simulink model "bd_par_auto2"  (Simulink 4.1.1)
settings: Solver=ode1  SolverMode=SingleTasking  StartTime=0.0  StopTime=max(cyc_mph(:,1))  FixedStep=1  MaxStep=1  RelTol=1e-3  AbsTol=1e-3
undefined symbols (not defined in the file): air_cp, amb_tmp, cs_charge_deplete_bool, cs_charge_trq, cs_electric_decel_spd, cs_electric_launch_spd_hi, cs_electric_launch_spd_lo, cs_hi_soc, cs_lo_soc, cs_min_trq_frac, cs_off_trq_frac, cyc_avg_time, cyc_cargo_mass, cyc_elevation_init, cyc_filter_bool, cyc_grade, cyc_mph, enable_stop, ess_cap_scale, ess_coulombic_eff, ess_init_soc, ess_max_ah_cap, ess_max_volts, ess_min_volts, ess_mod_airflow, ess_mod_cp, ess_mod_init_tmp, ess_module_mass, ess_module_num, ess_on, ess_res_scale_coef, ess_res_scale_fun, ess_set_tmp, ess_th_calc, ess_th_res_off, ess_th_res_on, ess_tmp, ess_voc, ex_calc, fc_ct_trq, fc_emis, fc_inertia, fc_map_spd, fc_max_trq, fc_on, fc_spd_scale, fc_trq_scale, fc_tstat, fd_inertia, fd_loss, fd_ratio, gb_dnshift_load, gb_dnshift_spd, gb_gears_num, gb_inertia, gb_num_init, gb_ratio, gb_shift_delay, gb_spd_scale, gb_trq_scale ... (+56)
libraries: lib_wheel2 x12, lib_accessory2 x3, lib_etc x2, lib_drive_cycle2 x1, lib_interactive x1, lib_drive_cycle x1, lib_exhaust x1, lib_fuel_converter3 x1
(part 17 of 18)

== system bd_par_auto2/fuel converter <fc>/IC Engine Model  &  Interface/ic engine model/engine torque/T_max ==
  w_APU : Inport  Port=1  LatchInput=off
  Saturation1 : Saturate  UpperLimit=max(fc_map_spd)*fc_spd_scale  LowerLimit=min(fc_map_spd)*fc_spd_scale  LinearizeAsGain=on
  max_torque lookup : Lookup  InputValues=fc_map_spd*fc_spd_scale  OutputValues=fc_max_trq*fc_trq_scale
  T_max : Outport  Port=1  InitialOutput=0
  tag scope: engine_speed=scoped
  wires:
  w_APU/1 -> Saturation1/1
  max_torque lookup/1 -> T_max/1
  Saturation1/1 -> max_torque lookup/1, [engine_speed]

== system bd_par_auto2/fuel converter <fc>/IC Engine Model  &  Interface/ic engine model/engine torque/effect of inertia (Nm) ==
  engine spd (rad/s) : Inport  Port=1  LatchInput=off
  >=0 : Saturate  UpperLimit=inf  LowerLimit=0  LinearizeAsGain=on
  Block NOTES : Subsystem
      settings: RTWFcnNameOpts=Auto  RTWFileNameOpts=Auto
      mask Display: disp('Block\nNOTES')
  Clock : Clock
      settings: DisplayTime=off  Decimation=10
  Constant : Constant  Orientation=left  Value=fc_inertia
  Constant1 : Constant  Value=max(fc_max_trq)*fc_trq_scale
  Constant2 : Constant  Orientation=left  Value=0.01
  Memory : Memory  X0=-0.1  InheritSampleTime=off
      settings: RTWStateStorageClass=Auto
  Memory1 : Memory  X0=vc_idle_spd*vc_key_on(1,2)  InheritSampleTime=off
      settings: RTWStateStorageClass=Auto
  MinMax : MinMax  Function=min  Inputs=2
  Product : Product  Inputs=2  Multiplication=Element-wise(.*)  SaturateOnIntegerOverflow=on
  Product1 : Product  Inputs=*/*  Multiplication=Element-wise(.*)  SaturateOnIntegerOverflow=on
  Relational : RelationalOperator  Operator=>
  Sum : Sum  Inputs=+-  SaturateOnIntegerOverflow=on
  Sum1 : Sum  Inputs=+-  SaturateOnIntegerOverflow=on
  Sum2 : Sum  Inputs=-+  SaturateOnIntegerOverflow=on
  Switch : Switch  Threshold=eps
  engine inertia as a function of total vehicle inertia (generous approximation) : Subsystem  Orientation=down
      settings: RTWFcnNameOpts=Auto  RTWFileNameOpts=Auto
  (Nm) : Outport  Port=1  InitialOutput=0
  wires:
  Sum/1 -> >=0/1, Switch/3
  Memory1/1 -> Sum/2
  Product/1 -> MinMax/1
  Constant1/1 -> Product/2
  engine inertia as a function of total vehicle inertia (generous approximation)/1(Out1) -> Product/1
  Product1/1 -> MinMax/2
  MinMax/1 -> (Nm)/1
  [cyc_mph_r_prev] -> Sum2/2
  [mpha_prev] -> Sum2/1
  Switch/1 -> Product1/1
  Sum1/1 -> Product1/2
  Constant/1 -> Product1/3
  Memory/1 -> Sum1/2
  Clock/1 -> Memory/1, Sum1/1
  Relational/1 -> Switch/2
  >=0/1 -> Switch/1
  Sum2/1 -> Relational/1
  Constant2/1 -> Relational/2
  engine spd (rad/s)/1 -> Memory1/1, Sum/1

== system bd_par_auto2/gearbox <gb> old/gearbox model & interface/gearbox model/Pout/Pin neglecting inertia/Pout/Pin (neglecting inertia) ==
  in_1 : Inport  Port=1  LatchInput=off
  in_2 : Inport  Port=2  LatchInput=off
  Fcn : Fcn  Expr=1/u
  Product : Product  Inputs=2  Multiplication=Element-wise(.*)  SaturateOnIntegerOverflow=on
  out_1 : Outport  Port=1  InitialOutput=0
  wires:
  in_1/1 -> Product/1
  Fcn/1 -> Product/2
  Product/1 -> out_1/1
  in_2/1 -> Fcn/1

== system bd_par_auto2/gearbox <gb> old/gearbox model & interface/gearbox model/Pout/Pin neglecting inertia/make division bombproof ==
  note: only add eps if Tin-Tinertia is == 0 (this avoids problems when Tin-Tineratia == -eps
      | which happens from time to time
  Tin-Tinertia : Inport  Port=1  LatchInput=off
  Block NOTES : Subsystem
      settings: RTWFcnNameOpts=Auto  RTWFileNameOpts=Auto
      mask Display: disp('Block\nNOTES')
  Constant : Constant  Orientation=up  Value=eps
  Constant1 : Constant  Orientation=up  Value=0
  Product : Product  Inputs=2  Multiplication=Element-wise(.*)  SaturateOnIntegerOverflow=on
  Relational Operator1 : RelationalOperator  Operator===
  make division bombproof : Sum  Inputs=++  SaturateOnIntegerOverflow=on
  Out1 : Outport  Port=1
  wires:
  Tin-Tinertia/1 -> make division bombproof/1, Relational Operator1/1
  Constant1/1 -> Relational Operator1/2
  Product/1 -> make division bombproof/2
  Relational Operator1/1 -> Product/1
  Constant/1 -> Product/2
  make division bombproof/1 -> Out1/1

== system bd_par_auto2/gearbox <gb> old/gearbox model & interface/gearbox model/gearbox controller interface/enhancedToWorkspace1 ==
  In1 : Inport  Port=1  LatchInput=off
  Terminator : Terminator
  wires:
  In1/1 -> Terminator/1

== system bd_par_auto2/gearbox <gb> old/gearbox model & interface/gearbox model/gearbox controller interface/enhancedToWorkspace8 ==
  In1 : Inport  Port=1  LatchInput=off
  Terminator : Terminator
  wires:
  In1/1 -> Terminator/1

== system bd_par_auto2/gearbox <gb> old/gearbox model & interface/gearbox model/loss (Nm)/3D discrete lookup table (sfun) ==
  lookup speed (rad/s) : Inport  Port=1  LatchInput=off
  lookup trq (Nm) : Inport  Port=2  LatchInput=off
  "gear_number  (e.g., 1, 2, 3)" : Inport  Port=3  LatchInput=off
  Mux : Mux  Inputs=3
  Saturation : Saturate  UpperLimit=max(tx_map_spd)  LowerLimit=min(tx_map_spd)  LinearizeAsGain=on
  Saturation1 : Saturate  UpperLimit=max(tx_map_trq)  LowerLimit=min(tx_map_trq)  LinearizeAsGain=on
  Saturation2 : Saturate  UpperLimit=size(tx_eff_map,3)  LowerLimit=1  LinearizeAsGain=on
  discrete interp2d : S-Function  FunctionName=sfun_discreteLookup3d  Parameters=tx_map_trq, tx_map_spd, tx_eff_map  PortCounts=[]  SFunctionModules=''
  tx_eff : Outport  Port=1
  wires:
  Saturation2/1 -> Mux/3
  "gear_number  (e.g., 1, 2, 3)"/1 -> Saturation2/1
  Saturation1/1 -> Mux/2
  lookup trq (Nm)/1 -> Saturation1/1
  Saturation/1 -> Mux/1
  lookup speed (rad/s)/1 -> Saturation/1
  Mux/1 -> discrete interp2d/1
  discrete interp2d/1 -> tx_eff/1

== system bd_par_auto2/gearbox <gb> old/gearbox model & interface/gearbox model/loss (Nm)/Block NOTES ==
  note: Revision Notes:
  note: 09/20/02:tm modifed lower input to switch after T_loss_at_input to pass the
      | total torque input as the loss when tx_eff=0
      | 5 July 2001:mpo changing loss block to a lookup table methodology
      | 12/20/00:tm revised loss saturation block. lower limit changed
      | from 1 to 0 and upper limit changed from 100 to inf to prevent over or under penalties

== system bd_par_auto2/gearbox <gb> old/gearbox model & interface/gearbox model/loss (Nm)/enhancedToWorkspace ==
  In1 : Inport  Port=1  LatchInput=off
  Terminator : Terminator
  wires:
  In1/1 -> Terminator/1

== system bd_par_auto2/hydraulic torque converter <htc> HEV/HTC for parallel HEV and Interface/model for parallel HEV/SR/K_adv ==
  "Req'd output trq and spd (Nm), (rad/s)" : Inport  Port=1  LatchInput=off
  >0 : Saturate  UpperLimit=inf  LowerLimit=eps  LinearizeAsGain=on
  K_adv=wout/(Tout)^0.5 : Fcn  Expr=u[2]/u[1]^0.5
  Saturation : Saturate  UpperLimit=max(htc_k_adv)  LowerLimit=min(htc_k_adv)  LinearizeAsGain=on
  K_adv : Outport  Port=1
  wires:
  Saturation/1 -> K_adv/1
  K_adv=wout/(Tout)^0.5/1 -> Saturation/1
  "Req'd output trq and spd (Nm), (rad/s)"/1 -> >0/1
  >0/1 -> K_adv=wout/(Tout)^0.5/1

== system bd_par_auto2/hydraulic torque converter <htc> HEV/HTC for parallel HEV and Interface/model for parallel HEV/SR/K_adv_coast ==
  "Req'd output trq and spd (Nm), (rad/s)" : Inport  Port=1  LatchInput=off
  K_adv=wout/(abs(Tout))^0.5 : Fcn  Expr=u[2]/abs(u[1]+eps)^0.5
  Saturation : Saturate  UpperLimit=max(htc_k_adv_coast)  LowerLimit=0  LinearizeAsGain=on
  K_adv_coast : Outport  Port=1
  wires:
  "Req'd output trq and spd (Nm), (rad/s)"/1 -> K_adv=wout/(abs(Tout))^0.5/1
  Saturation/1 -> K_adv_coast/1
  K_adv=wout/(abs(Tout))^0.5/1 -> Saturation/1

== system bd_par_auto2/hydraulic torque converter <htc> HEV/HTC for parallel HEV and Interface/model for parallel HEV/SR/enhancedToWorkspace ==
  In1 : Inport  Port=1  LatchInput=off
  To Workspace : ToWorkspace  VariableName=htc_locked  SampleTime=-1  SaveFormat=Array
  wires:
  In1/1 -> To Workspace/1

== system bd_par_auto2/hydraulic torque converter <htc> HEV/HTC for parallel HEV and Interface/model for parallel HEV/SR/enhancedToWorkspace1 ==
  In1 : Inport  Port=1  LatchInput=off
  To Workspace : ToWorkspace  VariableName=htc_coasting  SampleTime=-1  SaveFormat=Array
  wires:
  In1/1 -> To Workspace/1

== system bd_par_auto2/hydraulic torque converter <htc> HEV/HTC for parallel HEV and Interface/model for parallel HEV/SR/shifting SR ==
  T,w req out : Inport  Port=1  LatchInput=off
  w in : Inport  Port=2  LatchInput=off
  SR : Inport  Port=3  LatchInput=off
  -3200 rpm/second allowable in engine speed : Gain  Gain=-3200*pi/30  Multiplication=Element-wise(K.*u)  SaturateOnIntegerOverflow=on
  >0 : Saturate  UpperLimit=inf  LowerLimit=eps  LinearizeAsGain=on
  Clock : Clock
      settings: DisplayTime=off  Decimation=10
  Memory3 : Memory  X0=eps  InheritSampleTime=off
      settings: RTWStateStorageClass=Auto
  Memory4 : Memory  X0=0  InheritSampleTime=off
      settings: RTWStateStorageClass=Auto
  MinMax : MinMax  Function=min  Inputs=2
  SRmax= wout/win,min : Product  Inputs=*/  Multiplication=Element-wise(.*)  SaturateOnIntegerOverflow=on
  dt=t-(t-1) : Sum  Inputs=+-  SaturateOnIntegerOverflow=on
  "shifting, then limit  engine speed change" : Switch  Threshold=eps
  win,min= win,prev+rate*dt : Sum  Inputs=++  SaturateOnIntegerOverflow=on
  wout,req : Selector  InputType=Vector  ElementSrc=Internal  Elements=2  RowSrc=Internal  Rows=1  ColumnSrc=Internal  Columns=1  InputPortWidth=2
  SR limited : Outport  Port=1  InitialOutput=0
  wires:
  Memory4/1 -> dt=t-(t-1)/2
  Clock/1 -> Memory4/1, dt=t-(t-1)/1
  dt=t-(t-1)/1 -> -3200 rpm/second allowable in engine speed/1
  Memory3/1 -> win,min= win,prev+rate*dt/1
  win,min= win,prev+rate*dt/1 -> SRmax= wout/win,min/2
  wout,req/1 -> SRmax= wout/win,min/1
  T,w req out/1 -> wout,req/1
  [shifting] -> "shifting, then limit  engine speed change"/2
  SRmax= wout/win,min/1 -> MinMax/1
  SR/1 -> "shifting, then limit  engine speed change"/3, MinMax/2
  "shifting, then limit  engine speed change"/1 -> SR limited/1
  MinMax/1 -> "shifting, then limit  engine speed change"/1
  w in/1 -> >0/1
  >0/1 -> Memory3/1
  -3200 rpm/second allowable in engine speed/1 -> win,min= win,prev+rate*dt/2

== system bd_par_auto2/hydraulic torque converter <htc> HEV/HTC for parallel HEV and Interface/model for parallel HEV/T, shifting/T_max ==
  w_APU : Inport  Port=1  LatchInput=off
  TR : Inport  Port=2  LatchInput=off
  Block NOTES : Subsystem
      settings: RTWFcnNameOpts=Auto  RTWFileNameOpts=Auto
      mask Display: disp('Block\nNOTES')
  Constant : Constant  Value=1
  Gain : Gain  Gain=tc_mc_to_fc_ratio  Multiplication=Element-wise(K.*u)  SaturateOnIntegerOverflow=on
  Gain1 : Gain  Gain=tc_mc_to_fc_ratio  Multiplication=Element-wise(K.*u)  SaturateOnIntegerOverflow=on
  Saturation1 : Saturate  UpperLimit=max(fc_map_spd)*fc_spd_scale  LowerLimit=min(fc_map_spd)*fc_spd_scale  LinearizeAsGain=on
  Sum : Sum  Inputs=++  SaturateOnIntegerOverflow=on
  Switch : Switch  Threshold=eps
  Tin*TR= Tout : Product  Inputs=2  Multiplication=Element-wise(.*)  SaturateOnIntegerOverflow=on
  max_torque  mc lookup1 : Lookup  InputValues=mc_map_spd*mc_spd_scale  OutputValues=mc_max_trq*mc_overtrq_factor*mc_trq_scale
  max_torque lookup : Lookup  InputValues=fc_map_spd*fc_spd_scale  OutputValues=fc_max_trq*fc_trq_scale
  T_max max gain from htc : Outport  Port=1  InitialOutput=0
  wires:
  w_APU/1 -> Saturation1/1
  Tin*TR= Tout/1 -> T_max max gain from htc/1
  TR/1 -> Tin*TR= Tout/2
  max_torque lookup/1 -> Sum/1
  Saturation1/1 -> max_torque lookup/1, Gain/1
  Gain/1 -> max_torque  mc lookup1/1
  max_torque  mc lookup1/1 -> Gain1/1
  Constant/1 -> Switch/2
  Sum/1 -> Switch/1
  Gain1/1 -> Sum/2, Switch/3
  Switch/1 -> Tin*TR= Tout/1

== system bd_par_auto2/hydraulic torque converter <htc> HEV/HTC for parallel HEV and Interface/model for parallel HEV/T, shifting/engine speed estimator ==
  htc_spd_in_a : Inport  Port=1  LatchInput=off
  Memory2 : Memory  X0=0  InheritSampleTime=off
      settings: RTWStateStorageClass=Auto
  Out1 : Outport  Port=1
  wires:
  htc_spd_in_a/1 -> Memory2/1
  Memory2/1 -> Out1/1

== system bd_par_auto2/motor/controller <mc>/motor model & interface/mc model/N-m drive torque per W input/Block NOTES ==
  note: This block determines the ratio of req'd rotor torque to req'd electrical input power,
      |  which is proportional to efficiency if the motor is providing torque.  This ratio is used
      | to compute actual rotor torque given some input power which may be different from
      | the req'd value.
      |
      | If the denominator, the req'd input power, is zero, this block outputs inf,
      | which is a flag used by the block .../rotor drive torque available (Nm).

== system bd_par_auto2/motor/controller <mc>/motor model & interface/mc model/effect of inertia (Nm)/Block NOTES ==
  note: Torque required to accelerate the motor's inertia is calculated from the rate of change
      | of mc_spd_out_a.  It is no greater than the product of the maximum motor torque and
      | the fractional contribution of the motor's inertia to the total vehicle inertia.

== system bd_par_auto2/motor/controller <mc>/motor model & interface/mc model/effect of inertia (Nm)/motor inertia as a function of total vehicle inertia (generous approximation) ==
  gear ratio : Inport  Orientation=down  Port=1  LatchInput=off
  Product : Product  Orientation=down  Inputs=*/  Multiplication=Element-wise(.*)  SaturateOnIntegerOverflow=on
  Sum : Sum  Orientation=down  Inputs=++|  SaturateOnIntegerOverflow=on
  engine inertia as a fraction of total vehicle inertia  (generous approximation)--denomenator : Fcn  Orientation=down  Expr=mc_inertia*u^2
  engine inertia as a fraction of total vehicle inertia  (generous approximation)--numerator : Fcn  Orientation=down  Expr=mc_inertia*u^2
  Out1 : Outport  Orientation=down  Port=1
  wires:
  Sum/1 -> Product/2
  engine inertia as a fraction of total vehicle inertia  (generous approximation)--denomenator/1 -> Sum/2
  [current_veh_mass] -> Sum/1
  gear ratio/1 -> engine inertia as a fraction of total vehicle inertia  (generous approximation)--denomenator/1, engine inertia as a fraction of total vehicle inertia  (generous approximation)--numerator/1
  Product/1 -> Out1/1
  engine inertia as a fraction of total vehicle inertia  (generous approximation)--numerator/1 -> Product/1

== system bd_par_auto2/motor/controller <mc>/motor model & interface/mc model/enforce torque limit/Block NOTES ==
  note: This block enforces the maximum torque production and absorption
      | capability limits of the motor.  It assumes that exactly as much torque
      | can be absorbed as can be produced at a given speed.

== system bd_par_auto2/motor/controller <mc>/motor model & interface/mc model/enforce torque limit/enhancedToWorkspace ==
  In1 : Inport  Port=1  LatchInput=off
  To Workspace : ToWorkspace  VariableName=mc_max_trq_vec  SampleTime=-1  SaveFormat=Array
  wires:
  In1/1 -> To Workspace/1

== system bd_par_auto2/motor/controller <mc>/motor model & interface/mc model/mc tmp/Block NOTES ==
  note: This block models the thermal behavior of a motor
      | and controller  with active fluid cooling.
      | The module is modeled as a single lumped thermal mass.
      | The fan is on whenever the battery temp is > the set temp.

== system bd_par_auto2/motor/controller <mc>/motor model & interface/mc model/mc tmp/mc coolant ==
  Tcl : Inport  Port=1  LatchInput=off
  "Qmc " : Inport  Port=2  LatchInput=off
  Enable : EnablePort  StatesWhenEnabling=reset
  Constant : Constant  Value=mc_tstat
  Product1 : Product  Inputs=2  Multiplication=Element-wise(.*)  SaturateOnIntegerOverflow=on
  Relational Operator : RelationalOperator  Operator=<=
  Qmc_clt : Outport  Port=1  OutputWhenDisabled=reset  InitialOutput=0
  wires:
  Tcl/1 -> Relational Operator/2
  Constant/1 -> Relational Operator/1
  "Qmc "/1 -> Product1/2
  Product1/1 -> Qmc_clt/1
  Relational Operator/1 -> Product1/1

== system bd_par_auto2/motor/controller <mc>/motor model & interface/mc model/motor controller logic interface/motor controller logic ==
  bus voltage  previous : Inport  Port=1  LatchInput=off
  req'd input power (W) : Inport  Port=2  LatchInput=off
  req'd output spd (rad/s) : Inport  Port=3  LatchInput=off
  shifting : Inport  Port=4  LatchInput=off
  Abs : Abs  SaturateOnIntegerOverflow=on
  Abs1 : Abs  SaturateOnIntegerOverflow=on
  Block NOTES : Subsystem
      settings: RTWFcnNameOpts=Auto  RTWFileNameOpts=Auto
      mask Display: disp('Block\nNOTES')
  Constant : Constant  Value=mc_max_crrnt
  Constant1 : Constant  Value=0.001
  Constant2 : Constant  Orientation=left  Value=0
  Logical Operator1 : Logic  Orientation=up  Operator=NOT  Inputs=1
  MinMax : MinMax  Function=min  Inputs=2
  Product1 : Product  Inputs=2  Multiplication=Element-wise(.*)  SaturateOnIntegerOverflow=on
  Relational Operator : RelationalOperator  Operator=<=
  Relational Operator2 : RelationalOperator  Operator===
  Sign : Subsystem
      settings: RTWFcnNameOpts=Auto  RTWFileNameOpts=Auto
      mask Type: Sign
      mask Description: y = sign(x)
      mask Help: Sign Function:\n\t\t\ty = 1 if x > 0\n\t\t\ty = 0 if x = 0\n\t\t\ty = -1 if x < 0
      mask Display: plot(-50,-50,50,50,[-50,50],[0,0],[0,0],[-50,50],[-40,0],[-30,-30],[0,40],[30,30])
  Switch : Switch  Threshold=eps
  current-limited power : Product  Inputs=2  Multiplication=Element-wise(.*)  SaturateOnIntegerOverflow=on
  true if motor should be shut down : Logic  Operator=OR  Inputs=2
  req'd input power (W)1 : Outport  Port=1  InitialOutput=0
  tag scope: mc_crrnt_limited=scoped
  wires:
  shifting/1 -> true if motor should be shut down/2
  Logical Operator1/1 -> Switch/2
  true if motor should be shut down/1 -> Logical Operator1/1
  bus voltage  previous/1 -> Product1/1
  Constant/1 -> Product1/2
  req'd input power (W)/1 -> Abs/1, Sign/1(in_1)
  Abs/1 -> MinMax/2
  Sign/1(out_1) -> current-limited power/2
  Constant2/1 -> Switch/3
  Switch/1 -> req'd input power (W)1/1
  current-limited power/1 -> Switch/1
  Product1/1 -> MinMax/1, Relational Operator2/1
  MinMax/1 -> current-limited power/1, Relational Operator2/2
  Relational Operator2/1 -> [mc_crrnt_limited]
  Relational Operator/1 -> true if motor should be shut down/1
  Constant1/1 -> Relational Operator/2
  req'd output spd (rad/s)/1 -> Abs1/1
  Abs1/1 -> Relational Operator/1

== system bd_par_auto2/motor/controller <mc>/motor model & interface/mc model/motor speed estimator/Block NOTES ==
  note: The requested motor speed is replaced by an estimate of the
      | motor's previous speed, for loss and max. torque calculations,
      | whenever the vehicle missed the trace by more than 1 mph
      | on the last time step.

== system bd_par_auto2/motor/controller <mc>/motor model & interface/mc model/motor speed estimator/enhancedToWorkspace ==
  In1 : Inport  Port=1  LatchInput=off
  To Workspace : ToWorkspace  VariableName=mc_spd_est  SampleTime=-1  SaveFormat=Array
  wires:
  In1/1 -> To Workspace/1

== system bd_par_auto2/motor/controller <mc>/motor model & interface/mc model/motor speed estimator/init via port ==
  signal in : Inport  Port=1  LatchInput=off
  signal init : Inport  Port=2  LatchInput=off
  Constant : Constant  Value=1
  IC : InitialCondition  Value=0
  Switch : Switch  Threshold=0.5
  signal out : Outport  Port=1
  wires:
  signal init/1 -> Switch/3
  Switch/1 -> signal out/1
  IC/1 -> Switch/2
  Constant/1 -> IC/1
  signal in/1 -> Switch/1

== system bd_par_auto2/motor/controller <mc>/motor model & interface/mc model/rotor drive torque available (Nm)/Block NOTES ==
  note: This block computes the actual rotor torque given the actual motor input power and
      | the ratio (req'd rotor torque)/(req'd input power).
      |
      | If the above ratio has the value inf, which implies that the req'd input power is zero,
      | then the actual rotor torque is assumed to be zero.  This is not reflective of reality, of course:
      | with zero input power, the rotor torque would be the motor spin-loss torque at the given speed.
      | Because this simplification occurs only when req'd input power is zero, it does not.
      | affect fuel economy or max effort acceleration calculations.

== system bd_par_auto2/vehicle, wheel, & axle front/rear <wh> 2 axle --> 1 driveline/models and interface/vehicle <veh>/power logging--achieved/Joules ==
  In1 : Inport  Port=1  LatchInput=off
  To Workspace : ToWorkspace  VariableName=veh_energy_a  SampleTime=-1  SaveFormat=Array
  wires:
  In1/1 -> To Workspace/1

== system bd_par_auto2/vehicle, wheel, & axle front/rear <wh> 2 axle --> 1 driveline/models and interface/vehicle <veh>/power logging--achieved/horse power ==
  In1 : Inport  Port=1  LatchInput=off
  To Workspace : ToWorkspace  VariableName=veh_pwr_a_hp  SampleTime=-1  SaveFormat=Array
  wires:
  In1/1 -> To Workspace/1

== system bd_par_auto2/vehicle, wheel, & axle front/rear <wh> 2 axle --> 1 driveline/models and interface/vehicle <veh>/power logging--achieved/watts ==
  In1 : Inport  Port=1  LatchInput=off
  To Workspace : ToWorkspace  VariableName=veh_pwr_a  SampleTime=-1  SaveFormat=Array
  wires:
  In1/1 -> To Workspace/1

== system bd_par_auto2/vehicle, wheel, & axle front/rear <wh> 2 axle --> 1 driveline/models and interface/vehicle <veh>/power logging--request/Joules ==
  In1 : Inport  Port=1  LatchInput=off
  To Workspace : ToWorkspace  VariableName=veh_energy_r  SampleTime=-1  SaveFormat=Array
  wires:
  In1/1 -> To Workspace/1

== system bd_par_auto2/vehicle, wheel, & axle front/rear <wh> 2 axle --> 1 driveline/models and interface/vehicle <veh>/power logging--request/horse power ==
  In1 : Inport  Port=1  LatchInput=off
  To Workspace : ToWorkspace  VariableName=veh_pwr_r_hp  SampleTime=-1  SaveFormat=Array
  wires:
  In1/1 -> To Workspace/1

== system bd_par_auto2/vehicle, wheel, & axle front/rear <wh> 2 axle --> 1 driveline/models and interface/vehicle <veh>/power logging--request/watts ==
  In1 : Inport  Port=1  LatchInput=off
  To Workspace : ToWorkspace  VariableName=veh_pwr_r  SampleTime=-1  SaveFormat=Array
  wires:
  In1/1 -> To Workspace/1

== system bd_par_auto2/vehicle, wheel, & axle front/rear <wh> 2 axle --> 1 driveline/models and interface/vehicle <veh>/record achieved force outputs/enhancedToWorkspace ==
  In1 : Inport  Port=1  LatchInput=off
  To Workspace : ToWorkspace  VariableName=veh_pwr_accel_a  SampleTime=-1  SaveFormat=Array
  wires:
  In1/1 -> To Workspace/1

== system bd_par_auto2/vehicle, wheel, & axle front/rear <wh> 2 axle --> 1 driveline/models and interface/vehicle <veh>/record achieved force outputs/enhancedToWorkspace1 ==
  In1 : Inport  Port=1  LatchInput=off
  To Workspace : ToWorkspace  VariableName=veh_pwr_drag_a  SampleTime=-1  SaveFormat=Array
  wires:
  In1/1 -> To Workspace/1

== system bd_par_auto2/vehicle, wheel, & axle front/rear <wh> 2 axle --> 1 driveline/models and interface/vehicle <veh>/record achieved force outputs/enhancedToWorkspace2 ==
  In1 : Inport  Port=1  LatchInput=off
  To Workspace : ToWorkspace  VariableName=veh_pwr_ascent_a  SampleTime=-1  SaveFormat=Array
  wires:
  In1/1 -> To Workspace/1

== system bd_par_auto2/vehicle, wheel, & axle front/rear <wh> 2 axle --> 1 driveline/models and interface/vehicle <veh>/record achieved force outputs/enhancedToWorkspace3 ==
  In1 : Inport  Port=1  LatchInput=off
  To Workspace : ToWorkspace  VariableName=veh_pwr_rr_a  SampleTime=-1  SaveFormat=Array
  wires:
  In1/1 -> To Workspace/1

== system bd_par_auto2/vehicle, wheel, & axle front/rear <wh> 2 axle --> 1 driveline/models and interface/vehicle <veh>/record achieved force outputs/rolling resistance force ==
  average vehicle speed over time step (m/s) : Inport  Port=1  LatchInput=off
  force req'd to overcome rolling resistance (N) : lib_wheel2/Submodels/force req'd to overcome rolling resistance (N)
      settings: RTWFcnNameOpts=Auto  RTWFileNameOpts=Auto
  Fr (N) : Outport  Port=1
  wires:
  average vehicle speed over time step (m/s)/1 -> force req'd to overcome rolling resistance (N)/1
  force req'd to overcome rolling resistance (N)/1 -> Fr (N)/1

== system bd_par_auto2/vehicle, wheel, & axle front/rear <wh> 2 axle --> 1 driveline/models and interface/wheel and axle  front/rear <wh>/front force/brake request  controller interface ==
  F_front_brake_req : Outport  Port=1  InitialOutput=0
  wires:
  [F_front_brake_req] -> F_front_brake_req/1

== system bd_par_auto2/vehicle, wheel, & axle front/rear <wh> 2 axle --> 1 driveline/models and interface/wheel and axle  front/rear <wh>/front force/enhancedToWorkspace11 ==
  In1 : Inport  Port=1  LatchInput=off
  To Workspace : ToWorkspace  VariableName=wh_front_brake_r  SampleTime=-1  SaveFormat=Array
  wires:
  In1/1 -> To Workspace/1

== system bd_par_auto2/vehicle, wheel, & axle front/rear <wh> 2 axle --> 1 driveline/models and interface/wheel and axle  front/rear <wh>/limits and losses diagnostics/enhancedToWorkspace ==
  In1 : Inport  Port=1  LatchInput=off
  To Workspace : ToWorkspace  VariableName=wh_brake_loss_pwr  SampleTime=-1  SaveFormat=Array
  wires:
  In1/1 -> To Workspace/1

== system bd_par_auto2/vehicle, wheel, & axle front/rear <wh> 2 axle --> 1 driveline/models and interface/wheel and axle  front/rear <wh>/rear force/brake request controller interface1 ==
  F_rear_brake_req : Outport  Port=1  InitialOutput=0
  wires:
  [F_rear_brake_req] -> F_rear_brake_req/1

== system bd_par_auto2/vehicle, wheel, & axle front/rear <wh> 2 axle --> 1 driveline/models and interface/wheel and axle  front/rear <wh>/rear force/enhancedToWorkspace ==
  In1 : Inport  Port=1  LatchInput=off
  To Workspace : ToWorkspace  VariableName=wh_rear_brake_r  SampleTime=-1  SaveFormat=Array
  wires:
  In1/1 -> To Workspace/1

== system bd_par_auto2/vehicle, wheel, & axle front/rear <wh> 2 axle --> 1 driveline/models and interface/wheel and axle  front/rear <wh>/tire slip model (m/s)/Block NOTES ==
  note: This block implements the effects of finite tire slip (with respect to the road) on the
      | vehicle speed/wheel speed relationship.  Slip is defined as s=(omega*r - v) / v.  The
      | one-to-one mapping of slip to normalized tractive force, F_tract/W_front_axle, up to
      | the maximum, is stored in the variables "wh_slip" and "wh_slip_force_coeff."  The
      | slip calculation here is overridden if the actual axle speed and the requested axle
      | speed are the same, indicating that no drivetrain speed limits were encountered.

== system bd_par_auto2/vehicle, wheel, & axle front/rear <wh> 2 axle --> 1 driveline/models and interface/wheel and axle  front/rear <wh>/tire slip model (m/s)/front axle ==
  In1 : Inport  Port=1  LatchInput=off
  In2 : Inport  Port=2  LatchInput=off
  Abs : Abs  SaturateOnIntegerOverflow=on
  Constant3 : Constant  Orientation=up  Value=0
  F/W : Product  Inputs=*/  Multiplication=Element-wise(.*)  SaturateOnIntegerOverflow=on
  Product : Product  Inputs=2  Multiplication=Element-wise(.*)  SaturateOnIntegerOverflow=on
  Relational Operator : RelationalOperator  Orientation=up  Operator=~=
  Saturation : Saturate  UpperLimit=max(wh_slip_force_coeff)  LowerLimit=min(wh_slip_force_coeff)  LinearizeAsGain=on
  Sign : Signum
  Switch : Switch  Threshold=0
  s=s(F/W) : Lookup  InputValues=wh_slip_force_coeff  OutputValues=wh_slip
  Out1 : Outport  Port=1
  wires:
  Product/1 -> Out1/1
  In1/1 -> F/W/2
  In2/1 -> Sign/1, Abs/1
  s=s(F/W)/1 -> Product/1
  Sign/1 -> Product/2
  F/W/1 -> Switch/1
  Switch/1 -> Saturation/1
  Saturation/1 -> s=s(F/W)/1
  Abs/1 -> Relational Operator/1, F/W/1
  Relational Operator/1 -> Switch/2
  Constant3/1 -> Relational Operator/2, Switch/3

== system bd_par_auto2/vehicle, wheel, & axle front/rear <wh> 2 axle --> 1 driveline/models and interface/wheel and axle  front/rear <wh>/tire slip model (m/s)/rear axle ==
  In1 : Inport  Port=1  LatchInput=off
  In2 : Inport  Port=2  LatchInput=off
  Abs : Abs  SaturateOnIntegerOverflow=on
  Constant3 : Constant  Orientation=up  Value=0
  F/W : Product  Inputs=*/  Multiplication=Element-wise(.*)  SaturateOnIntegerOverflow=on
  Product : Product  Inputs=2  Multiplication=Element-wise(.*)  SaturateOnIntegerOverflow=on
  Relational Operator : RelationalOperator  Orientation=up  Operator=~=
  Saturation : Saturate  UpperLimit=max(wh_slip_force_coeff)  LowerLimit=min(wh_slip_force_coeff)  LinearizeAsGain=on
  Sign : Signum
  Switch : Switch  Threshold=0
  s=s(F/W) : Lookup  InputValues=wh_slip_force_coeff  OutputValues=wh_slip
  Out1 : Outport  Port=1
  wires:
  Product/1 -> Out1/1
  In1/1 -> F/W/2
  In2/1 -> Sign/1, Abs/1
  s=s(F/W)/1 -> Product/1
  Sign/1 -> Product/2
  F/W/1 -> Switch/1
  Switch/1 -> Saturation/1
  Saturation/1 -> s=s(F/W)/1
  Abs/1 -> Relational Operator/1, F/W/1
  Relational Operator/1 -> Switch/2
  Constant3/1 -> Relational Operator/2, Switch/3

== system bd_par_auto2/vehicle, wheel, & axle front/rear <wh> 2 axle --> 1 driveline/models and interface/wheel and axle  front/rear <wh>/tire slip model (rad/s)/enhancedToWorkspace ==
  In1 : Inport  Port=1  LatchInput=off
  To Workspace : ToWorkspace  VariableName=wh_slip_r  SampleTime=-1  SaveFormat=Array
  wires:
  In1/1 -> To Workspace/1

== system bd_par_auto2/vehicle, wheel, & axle front/rear <wh> 2 axle --> 1 driveline/models and interface/wheel and axle  front/rear <wh>/tire slip model (rad/s)/front slip ==
  In1 : Inport  Port=1  LatchInput=off
  In2 : Inport  Port=2  LatchInput=off
  Abs : Abs  SaturateOnIntegerOverflow=on
  F/W : Product  Inputs=*/  Multiplication=Element-wise(.*)  SaturateOnIntegerOverflow=on
  Product : Product  Inputs=2  Multiplication=Element-wise(.*)  SaturateOnIntegerOverflow=on
  Saturation : Saturate  UpperLimit=max(wh_slip_force_coeff)  LowerLimit=min(wh_slip_force_coeff)  LinearizeAsGain=on
  Sign : Signum
  s=s(F/W) : Lookup  InputValues=wh_slip_force_coeff  OutputValues=wh_slip
  Out1 : Outport  Port=1
  wires:
  Product/1 -> Out1/1
  In1/1 -> F/W/2
  s=s(F/W)/1 -> Product/1
  In2/1 -> Sign/1, Abs/1
  Sign/1 -> Product/2
  Abs/1 -> F/W/1
  F/W/1 -> Saturation/1
  Saturation/1 -> s=s(F/W)/1

== system bd_par_auto2/vehicle, wheel, & axle front/rear <wh> 2 axle --> 1 driveline/models and interface/wheel and axle  front/rear <wh>/tire slip model (rad/s)/rear slip ==
  In1 : Inport  Port=1  LatchInput=off
  In2 : Inport  Port=2  LatchInput=off
  Abs : Abs  SaturateOnIntegerOverflow=on
  F/W : Product  Inputs=*/  Multiplication=Element-wise(.*)  SaturateOnIntegerOverflow=on
  Product : Product  Inputs=2  Multiplication=Element-wise(.*)  SaturateOnIntegerOverflow=on
  Saturation : Saturate  UpperLimit=max(wh_slip_force_coeff)  LowerLimit=min(wh_slip_force_coeff)  LinearizeAsGain=on
  Sign : Signum
  s=s(F/W) : Lookup  InputValues=wh_slip_force_coeff  OutputValues=wh_slip
  Out1 : Outport  Port=1
  wires:
  Product/1 -> Out1/1
  In1/1 -> F/W/2
  s=s(F/W)/1 -> Product/1
  In2/1 -> Sign/1, Abs/1
  Sign/1 -> Product/2
  Abs/1 -> F/W/1
  F/W/1 -> Saturation/1
  Saturation/1 -> s=s(F/W)/1

== system bd_par_auto2/<cs> control strategy/Automatic Transmission  Control/gearbox control for automatic transmission/gearbox control for use w/ AT/downshift  command/load fraction ==
  In1 : Inport  Port=1  LatchInput=off
  S-Function : S-Function  FunctionName=sfun_gearbox  Parameters=load, spd  PortCounts=[]  SFunctionModules=''
  Out1 : Outport  Port=1  InitialOutput=0
  wires:
  In1/1 -> S-Function/1
  S-Function/1 -> Out1/1

== system bd_par_auto2/<cs> control strategy/Automatic Transmission  Control/gearbox control for automatic transmission/gearbox control for use w/ AT/downshift  command1/load fraction ==
  In1 : Inport  Port=1  LatchInput=off
  S-Function : S-Function  FunctionName=sfun_gearbox  Parameters=load, spd  PortCounts=[]  SFunctionModules=''
  Out1 : Outport  Port=1  InitialOutput=0
  wires:
  S-Function/1 -> Out1/1
  In1/1 -> S-Function/1

== system bd_par_auto2/<cs> control strategy/Automatic Transmission  Control/gearbox control for automatic transmission/gearbox control for use w/ AT/est. engine trq and spd/Block NOTES ==
  note: Estimate engine torque and speed associated with the previous gear, assuming that
      | the gearbox efficiency is constant.

== system bd_par_auto2/<cs> control strategy/Automatic Transmission  Control/gearbox control for automatic transmission/gearbox control for use w/ AT/est. engine trq and spd/K_adv ==
  "Req'd output trq and spd (Nm), (rad/s)" : Inport  Port=1  LatchInput=off
  K_adv=wout/(Tout)^0.5 : Fcn  Expr=u[2]/u[1]^0.5
  Saturation : Saturate  UpperLimit=max(htc_k_adv)  LowerLimit=min(htc_k_adv)  LinearizeAsGain=on
  Saturation2 : Saturate  UpperLimit=inf  LowerLimit=eps  LinearizeAsGain=on
  K_adv : Outport  Port=1
  wires:
  Saturation/1 -> K_adv/1
  K_adv=wout/(Tout)^0.5/1 -> Saturation/1
  Saturation2/1 -> K_adv=wout/(Tout)^0.5/1
  "Req'd output trq and spd (Nm), (rad/s)"/1 -> Saturation2/1

== system bd_par_auto2/<cs> control strategy/Automatic Transmission  Control/gearbox control for automatic transmission/gearbox control for use w/ AT/est. engine trq and spd assuming lockup/Block NOTES ==
  note: Estimate engine torque and speed associated with the current gear, assuming that
      | the gearbox efficiency is constant.

== system bd_par_auto2/<cs> control strategy/Automatic Transmission  Control/gearbox control for automatic transmission/gearbox control for use w/ AT/shifting1/time since last shift ==
  in_1 : Inport  Port=1  LatchInput=off
  just shifted : Subsystem
      settings: RTWFcnNameOpts=Auto  RTWFileNameOpts=Auto
      mask Display: disp('just\nshifted')
  timer : Subsystem
      settings: RTWFcnNameOpts=Auto  RTWFileNameOpts=Auto
      mask Display: disp('timer')
  out_1 : Outport  Port=1  InitialOutput=0
  wires:
  timer/1(time) -> out_1/1
  just shifted/1(out_1) -> timer/1(trigger)
  in_1/1 -> just shifted/1(in_1)

== system bd_par_auto2/<cs> control strategy/Automatic Transmission  Control/gearbox control for automatic transmission/gearbox control for use w/ AT/upshift  command/load fraction ==
  In1 : Inport  Port=1  LatchInput=off
  S-Function : S-Function  FunctionName=sfun_gearbox  Parameters=load, spd  PortCounts=[]  SFunctionModules=''
  Out1 : Outport  Port=1  InitialOutput=0
  wires:
  In1/1 -> S-Function/1
  S-Function/1 -> Out1/1

== system bd_par_auto2/<cs> control strategy/Clutch Control/Clutch Control/parallel clutch control/gearbox speed estimator/Block NOTES ==
  note: The requested engine speed is replaced by an estimate of the
      | engine's previous speed whenever the vehicle missed the trace
      |  by more than 1 mph on the last time step.

== system bd_par_auto2/<cs> control strategy/Clutch Control/Clutch Control/parallel clutch control/gearbox speed estimator/dt ==
  Clock : Clock
      settings: DisplayTime=off  Decimation=10
  Memory1 : Memory  X0=-1  InheritSampleTime=off
      settings: RTWStateStorageClass=Auto
  Sum4 : Sum  Inputs=+-  SaturateOnIntegerOverflow=on
  Out1 : Outport  Port=1  InitialOutput=0
  wires:
  Sum4/1 -> Out1/1
  Memory1/1 -> Sum4/2
  Clock/1 -> Memory1/1, Sum4/1

== system bd_par_auto2/ess config/energy storage <ess>/energy storage <ess>/Model/compute current/enhancedToWorkspace2 ==
  In1 : Inport  Port=1  LatchInput=off
  Terminator : Terminator
  wires:
  In1/1 -> Terminator/1

== system bd_par_auto2/ess config/energy storage <ess>/energy storage <ess>/Model/ess tmp/Block NOTES ==
  note: This block models the thermal behavior of a battery module with active air cooling.
      | The module is modeled as a single lumped thermal mass.
      | The fan is on whenever the battery temp is > the set temp.

== system bd_par_auto2/ess config/energy storage <ess>/energy storage <ess>/Model/ess tmp/Tair,ave ==
  Qess_case : Inport  Port=1  LatchInput=off
  Enable : EnablePort  StatesWhenEnabling=reset
  Block NOTES : Subsystem
      settings: RTWFcnNameOpts=Auto  RTWFileNameOpts=Auto
      mask Display: disp('Block\nNOTES')
  Tamb-(Q/mcp)/2 : Fcn  Expr=amb_tmp - (u(1)/(ess_mod_airflow*air_cp))/2
  do ex calcs?1 : Constant  Value=ess_th_res_on
  Tair_ave : Outport  Port=1  OutputWhenDisabled=reset  InitialOutput=amb_tmp
  Th Res : Outport  Port=2  OutputWhenDisabled=reset  InitialOutput=ess_th_res_off
  wires:
  Tamb-(Q/mcp)/2/1 -> Tair_ave/1
  Qess_case/1 -> Tamb-(Q/mcp)/2/1
  do ex calcs?1/1 -> Th Res/1

== system bd_par_auto2/ess config/energy storage <ess>/energy storage <ess>/Model/limit power/Limits ==
  SOC  high limited : Inport  Port=1  LatchInput=off
  not SOC  low limited : Inport  Port=2  LatchInput=off
  power req : Inport  Port=3  LatchInput=off
  power bat limited : Inport  Port=4  LatchInput=off
  V used : Inport  Port=5  LatchInput=off
  V mc_min_volts : Inport  Port=6  LatchInput=off
  V battery (.5Voc) : Inport  Port=7  LatchInput=off
  V ess_min_volts : Inport  Port=8  LatchInput=off
  Logical Operator1 : Logic  Operator=NOT  Inputs=1
  Relational Operator{1,3..5} (4 alike) : RelationalOperator  Operator===
  limited by battery : Logic  Operator=AND  Inputs=2
  limited by battery min V : Logic  Operator=AND  Inputs=2
  limited by motor controller : Logic  Operator=AND  Inputs=2
  tag scope: ess_minV_limited=scoped, ess_pwr_limited=scoped, ess_soc_hi_limited=scoped, ess_soc_low_limited=scoped, mc_voltage_limited=scoped
  wires:
  power bat limited/1 -> Relational Operator1/2
  V mc_min_volts/1 -> Relational Operator3/2
  V used/1 -> Relational Operator3/1, Relational Operator4/1, Relational Operator5/1
  V battery (.5Voc)/1 -> Relational Operator4/2
  V ess_min_volts/1 -> Relational Operator5/2
  limited by motor controller/1 -> [mc_voltage_limited]
  limited by battery/1 -> [ess_pwr_limited]
  limited by battery min V/1 -> [ess_minV_limited]
  Relational Operator3/1 -> limited by motor controller/2
  Relational Operator1/1 -> limited by motor controller/1, limited by battery/1, limited by battery min V/1
  Relational Operator4/1 -> limited by battery/2
  Relational Operator5/1 -> limited by battery min V/2
  power req/1 -> Relational Operator1/1
  Logical Operator1/1 -> [ess_soc_low_limited]
  not SOC  low limited/1 -> Logical Operator1/1
  SOC  high limited/1 -> [ess_soc_hi_limited]

== system bd_par_auto2/ess config/energy storage <ess>/energy storage <ess>/Model/max pack pwr (W)1/Rchg (ohms)1 ==
  x0 : Inport  Port=1  LatchInput=off
  y0 : Inport  Port=2  LatchInput=off
  Mux : Mux  Inputs=2
      settings: DisplayOption=none
  S-function : S-Function  FunctionName=sftable2  Parameters=xindex, yindex, table  PortCounts=[]  SFunctionModules=''
  table out : Outport  Port=1  InitialOutput=0
  wires:
  Mux/1 -> S-function/1
  x0/1 -> Mux/1
  S-function/1 -> table out/1
  y0/1 -> Mux/2

== system bd_par_auto2/ess config/energy storage <ess>/energy storage <ess>/Model/max pack pwr (W)1/Rdis (ohms) ==
  x0 : Inport  Port=1  LatchInput=off
  y0 : Inport  Port=2  LatchInput=off
  Mux : Mux  Inputs=2
      settings: DisplayOption=none
  S-function : S-Function  FunctionName=sftable2  Parameters=xindex, yindex, table  PortCounts=[]  SFunctionModules=''
  table out : Outport  Port=1  InitialOutput=0
  wires:
  Mux/1 -> S-function/1
  x0/1 -> Mux/1
  S-function/1 -> table out/1
  y0/1 -> Mux/2

== system bd_par_auto2/ess config/energy storage <ess>/energy storage <ess>/Model/max pack pwr (W)1/VOC (V) ==
  x0 : Inport  Port=1  LatchInput=off
  y0 : Inport  Port=2  LatchInput=off
  Mux : Mux  Inputs=2
      settings: DisplayOption=none
  S-function : S-Function  FunctionName=sftable2  Parameters=xindex, yindex, table  PortCounts=[]  SFunctionModules=''
  table out : Outport  Port=1  InitialOutput=0
  wires:
  Mux/1 -> S-function/1
  x0/1 -> Mux/1
  S-function/1 -> table out/1
  y0/1 -> Mux/2

== system bd_par_auto2/ess config/energy storage <ess>/energy storage <ess>/Model/pack Voc, Rint/Rchg (ohms) ==
  x0 : Inport  Port=1  LatchInput=off
  y0 : Inport  Port=2  LatchInput=off
  Mux : Mux  Inputs=2
      settings: DisplayOption=none
  S-function : S-Function  FunctionName=sftable2  Parameters=xindex, yindex, table  PortCounts=[]  SFunctionModules=''
  table out : Outport  Port=1  InitialOutput=0
  wires:
  y0/1 -> Mux/2
  S-function/1 -> table out/1
  x0/1 -> Mux/1
  Mux/1 -> S-function/1

== system bd_par_auto2/ess config/energy storage <ess>/energy storage <ess>/Model/pack Voc, Rint/Rdis (ohms) ==
  x0 : Inport  Port=1  LatchInput=off
  y0 : Inport  Port=2  LatchInput=off
  Mux : Mux  Inputs=2
      settings: DisplayOption=none
  S-function : S-Function  FunctionName=sftable2  Parameters=xindex, yindex, table  PortCounts=[]  SFunctionModules=''
  table out : Outport  Port=1  InitialOutput=0
  wires:
  y0/1 -> Mux/2
  S-function/1 -> table out/1
  x0/1 -> Mux/1
  Mux/1 -> S-function/1

== system bd_par_auto2/ess config/energy storage <ess>/energy storage <ess>/Model/pack Voc, Rint/VOC (V) ==
  x0 : Inport  Port=1  LatchInput=off
  y0 : Inport  Port=2  LatchInput=off
  Mux : Mux  Inputs=2
      settings: DisplayOption=none
  S-function : S-Function  FunctionName=sftable2  Parameters=xindex, yindex, table  PortCounts=[]  SFunctionModules=''
  table out : Outport  Port=1  InitialOutput=0
  wires:
  y0/1 -> Mux/2
  S-function/1 -> table out/1
  x0/1 -> Mux/1
  Mux/1 -> S-function/1

== system bd_par_auto2/fuel converter <fc>/IC Engine Model  &  Interface/ic engine model/engine speed estimator/no-lag Reset Integrator/dt ==
  Clock : Clock
      settings: DisplayTime=off  Decimation=10
  Memory1 : Memory  X0=-0.1  InheritSampleTime=off
      settings: RTWStateStorageClass=Auto
  Sum1 : Sum  Inputs=+-  SaturateOnIntegerOverflow=on
  out_1 : Outport  Port=1  InitialOutput=0
  wires:
  Sum1/1 -> out_1/1
  Memory1/1 -> Sum1/2
  Clock/1 -> Memory1/1, Sum1/1

== system bd_par_auto2/fuel converter <fc>/IC Engine Model  &  Interface/ic engine model/engine torque/effect of inertia (Nm)/Block NOTES ==
  note: Torque required to accelerate the engine inertia is taken from the engine
      | acceleration, and is assumed to be no less than zero if the trace was missed
      | at all on the previous time step.
      |
      | The torque required to accelerate the engine's inertia is never assumed to
      | be more than the product of the engine's maximum torque and the engine's
      | contribution to the total vehicle inertia.

== system bd_par_auto2/fuel converter <fc>/IC Engine Model  &  Interface/ic engine model/engine torque/effect of inertia (Nm)/engine inertia as a function of total vehicle inertia (generous approximation) ==
  Product : Product  Orientation=down  Inputs=*/  Multiplication=Element-wise(.*)  SaturateOnIntegerOverflow=on
  Sum : Sum  Orientation=down  Inputs=++|  SaturateOnIntegerOverflow=on
  engine inertia as a fraction of total vehicle inertia  (generous approximation)--denomenator : Fcn  Orientation=down  Expr=fc_inertia*(u*fd_ratio/wh_radius)^2
  engine inertia as a fraction of total vehicle inertia  (generous approximation)--numerator : Fcn  Orientation=down  Expr=fc_inertia*(u*fd_ratio/wh_radius)^2
  veh mass calc : Subsystem
      settings: RTWFcnNameOpts=Auto  RTWFileNameOpts=Auto
  Out1 : Outport  Orientation=down  Port=1
  wires:
  [gear_ratio] -> engine inertia as a fraction of total vehicle inertia  (generous approximation)--numerator/1, engine inertia as a fraction of total vehicle inertia  (generous approximation)--denomenator/1
  veh mass calc/1(Out1) -> Sum/1
  engine inertia as a fraction of total vehicle inertia  (generous approximation)--denomenator/1 -> Sum/2
  engine inertia as a fraction of total vehicle inertia  (generous approximation)--numerator/1 -> Product/1
  Sum/1 -> Product/2
  Product/1 -> Out1/1

== system bd_par_auto2/gearbox <gb> old/gearbox model & interface/gearbox model/Pout/Pin neglecting inertia/make division bombproof/Block NOTES ==
  note: this block added 10 July 2001 by mpo:
      | originally a -eps was added to the denominator by default.
      | However, cases were ecountered where Tin-Tineratia was equal to -eps causing
      | the denominator to be zero. This added checking is more rhobust

== system bd_par_auto2/hydraulic torque converter <htc> HEV/HTC for parallel HEV and Interface/model for parallel HEV/T, shifting/T_max/Block NOTES ==
  note: Notes: engine_on flag causes algebric loop. Is it necessary?
      | Doesn't seem to be. Disabled 10/31/00:tm

== system bd_par_auto2/motor/controller <mc>/motor model & interface/mc model/motor controller logic interface/motor controller logic/Block NOTES ==
  note: This block models a motor/controller's logic, modulating the power input requirement as follows:
      | - enforcing the maximum current limit of the motor/controller
      | - shutting the motor off if the average speed over the time step ==0
      | - shutting the motor off if the transmission is shifting.

== system bd_par_auto2/motor/controller <mc>/motor model & interface/mc model/motor controller logic interface/motor controller logic/Sign ==
  in_1 : Inport  Port=1  LatchInput=off
  Constant : Constant  Value=0
  Relational Operator : RelationalOperator  Operator=>
  Relational Operator1 : RelationalOperator  Operator=<
  Sum : Sum  Inputs=+-  SaturateOnIntegerOverflow=on
  out_1 : Outport  Port=1  InitialOutput=0
  wires:
  Sum/1 -> out_1/1
  Relational Operator/1 -> Sum/1
  Relational Operator1/1 -> Sum/2
  Constant/1 -> Relational Operator/2, Relational Operator1/2
  in_1/1 -> Relational Operator1/1, Relational Operator/1

== system bd_par_auto2/<cs> control strategy/Automatic Transmission  Control/gearbox control for automatic transmission/gearbox control for use w/ AT/shifting1/time since last shift/just shifted ==
  in_1 : Inport  Port=1  LatchInput=off
  Memory : Memory  X0=1  InheritSampleTime=off
      settings: RTWStateStorageClass=Auto
  Relational Operator : RelationalOperator  Operator=~=
  out_1 : Outport  Port=1  InitialOutput=0
  wires:
  in_1/1 -> Memory/1, Relational Operator/2
  Memory/1 -> Relational Operator/1
  Relational Operator/1 -> out_1/1

== system bd_par_auto2/<cs> control strategy/Automatic Transmission  Control/gearbox control for automatic transmission/gearbox control for use w/ AT/shifting1/time since last shift/timer ==
  trigger : Inport  Port=1  LatchInput=off
  Constant : Constant  Value=1
  Constant1 : Constant  Value=0
  Constant2 : Constant  Value=0
  Switch : Switch  Threshold=eps
  no-lag Reset Integrator : Subsystem  mask(No-lag Reset Integrator){@1=15}
      mask prompts: @1 "Initial Value"
      mask help: No-lag Reset Integrator
      mask init:
      | initval=@1;
      settings: RTWFcnNameOpts=Auto  RTWFileNameOpts=Auto
      mask Help: Integrates first input using Euler technique.\nAt the time step that input 2 <> zero,\noutput is reset to input 3.
      mask Display: disp('1/s\nw/ reset\nno lag')
  time : Outport  Port=1  InitialOutput=0
  wires:
  no-lag Reset Integrator/1(out_1) -> Switch/3
  Constant1/1 -> no-lag Reset Integrator/3(in_3)
  Constant/1 -> no-lag Reset Integrator/1(in_1)
  Constant2/1 -> Switch/1
  trigger/1 -> no-lag Reset Integrator/2(in_2), Switch/2
  Switch/1 -> time/1

== system bd_par_auto2/ess config/energy storage <ess>/energy storage <ess>/Model/ess tmp/Tair,ave/Block NOTES ==
  note: This block determins the average temperature of the cooling air over the module.

== system bd_par_auto2/fuel converter <fc>/IC Engine Model  &  Interface/ic engine model/engine torque/effect of inertia (Nm)/engine inertia as a function of total vehicle inertia (generous approximation)/veh mass calc ==
  Out1 : Outport  Port=1
  wires:
  [current_veh_mass] -> Out1/1

== system bd_par_auto2/<cs> control strategy/Automatic Transmission  Control/gearbox control for automatic transmission/gearbox control for use w/ AT/shifting1/time since last shift/timer/no-lag Reset Integrator ==
  in_1 : Inport  Port=1  LatchInput=off
  in_2 : Inport  Port=2  LatchInput=off
  in_3 : Inport  Port=3  LatchInput=off
  Constant : Constant  Orientation=up  Value=0
  Memory : Memory  Orientation=left  X0=initval  InheritSampleTime=off
      settings: RTWStateStorageClass=Auto
  Product : Product  Inputs=2  Multiplication=Element-wise(.*)  SaturateOnIntegerOverflow=on
  Sum : Sum  Inputs=++  SaturateOnIntegerOverflow=on
  Switch : Switch  Threshold=eps
  dt : Subsystem  Orientation=down
      settings: RTWFcnNameOpts=Auto  RTWFileNameOpts=Auto
  in_2==0 : RelationalOperator  Operator===
  out_1 : Outport  Port=1  InitialOutput=0
  wires:
  Constant/1 -> in_2==0/2
  in_2==0/1 -> Switch/2
  Switch/1 -> Memory/1, out_1/1
  Sum/1 -> Switch/1
  Memory/1 -> Sum/1
  Product/1 -> Sum/2
  dt/1(out_1) -> Product/1
  in_1/1 -> Product/2
  in_2/1 -> in_2==0/1
  in_3/1 -> Switch/3
